simulink model "springmassdamper"  (R2023a)
settings: Solver=VariableStepAuto  StartTime=0.0  StopTime=10  FixedStep=0.01  MaxStep=0.001  RelTol=1e-3
values from neighbouring files (symbols this model uses):
  b = 10    [spring_mass_damper.m]
  k = 400    [spring_mass_damper.m]
  m = massvalues(i)    [spring_mass_damper.m]
  x0 = 1    [spring_mass_damper.m]
settings Model: Creator=Mohamed Ezzelrgal  LastModifiedBy=Mohamed Ezzelrgal

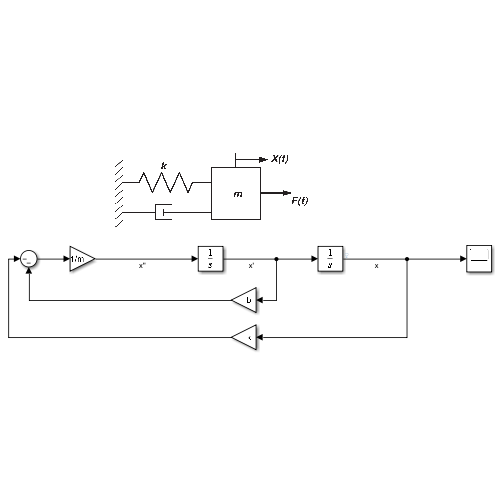
[thumbnail: Simulink's stored preview of the top-level diagram]
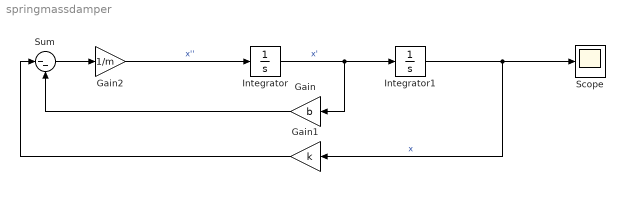
== system springmassdamper ==
  Gain : Gain  Gain=b
  Gain1 : Gain  Gain=k
  Gain2 : Gain  Gain=1/m
  Integrator : Integrator
  Integrator1 : Integrator  InitialCondition=x0
  Scope : Scope
  Sum : Sum  Inputs=|--
  wires:
  Gain2/1 -> Integrator/1  "x''"
  Integrator/1 -> Gain/1, Integrator1/1  "x'"
  Integrator1/1 -> Scope/1, Gain1/1  "x"
  Gain/1 -> Sum/2
  Gain1/1 -> Sum/1
  Sum/1 -> Gain2/1
